simulink model "LundellAlternatorDC"  (R2018a)
settings: Solver=VariableStepAuto  StartTime=0  StopTime=0.2  FixedStep=1e-6
undefined symbols (not defined in the file): alternator, i_f_max, n_r, rectifier, T_s, v_dc_ref
libraries: fl_lib x32, nesl_utility x31, elec_lib x20, powerlib_meascontrol x6, SimscapeCustomBlocks_lib x2
settings Model: Creator=gabrielrodrigues  LastModifiedBy=gabrielrodrigues
settings DataIOCC: ReturnWorkspaceOutputs=on
settings CodeAppCC: StateflowObjectComments=on
settings SimscapeCC: SimscapeNormalizeSystem=off  SimscapeLogType=local  SimscapeLogLimitData=off

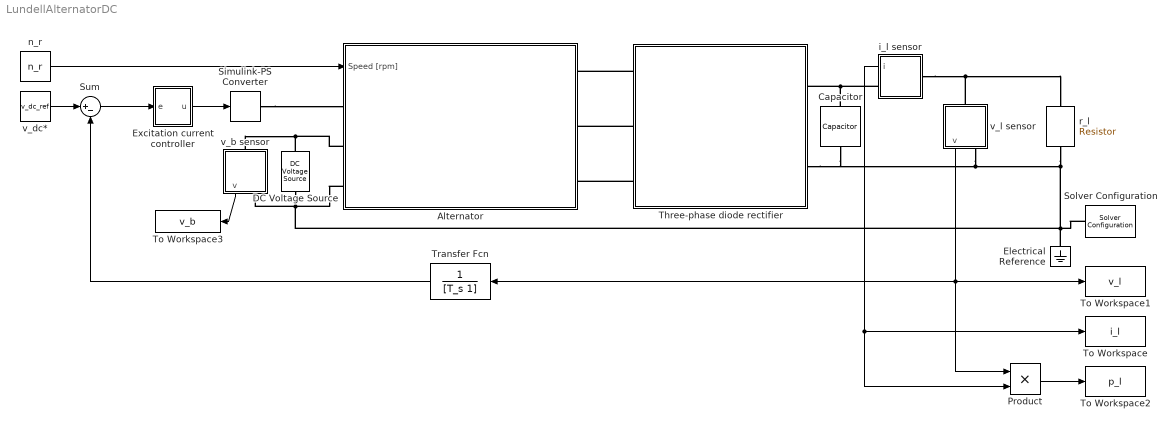
== system LundellAlternatorDC ==
  Alternator : Subsystem
  Capacitor : fl_lib/Electrical/Electrical Elements/Capacitor  c=rectifier.filter.c F  r=1e-6 Ohm  g=0 1/Ohm  i_specify=off  i_priority=None  i=0 A  i_nominal_specify=off  i_nominal_unit=A  i_nominal_value=1  v_specify=off  v_priority=None  v=0 V  v_nominal_specify=off  v_nominal_unit=V  v_nominal_value=1  vc_specify=off  vc_priority=High  vc=0 V  vc_nominal_specify=off  vc_nominal_unit=V  vc_nominal_value=1
  DC Voltage Source : elec_lib/Additional Components/SPICE-Compatible Components/Sources/DC Voltage Source  DC=i_f_max * alternator.rotor.r.value V
      settings: SourceProductName=Simscape Electronics  SourceProductBaseCode=SN
  Electrical Reference : fl_lib/Electrical/Electrical Elements/Electrical Reference
  Excitation current controller : Subsystem  mask{controller_on_off=Controller active}
      mask TypeOptions controller_on_off: Controller active | Controller bypassed
  Product : Product
  Simulink-PS Converter : nesl_utility/Simulink-PS Converter  PhysicalDomain=network_engine_domain  SubClassName=ps_input  LeftPortType=input  RightPortType=output  PseudoPeriodic=off  Frequencies=[]  NoiseDistribution=none  NoiseParameters=[]  Unit=1  AffineConversion=off  FilteringAndDerivatives=provide  SimscapeFilterOrder=1  InputFilterTimeConstant=0.001  UdotUserProvided=0
  Solver Configuration : nesl_utility/Solver Configuration  PhysicalDomain=network_engine_domain  SubClassName=solver  LeftPortType=input  RightPortType=generic  Tones=[]  Harmonics=[]  SimulateNoise=off  Profile=off  UseLocalSampling=off  EnableSwitchedLinearOptims=on  FrequencyDomain=off  UseCCode=off  RelTol=0.001  AbsTol=1e-06  MinStep=1e-09  ToWorkspace=off  RevertToSquareIcSolve=off  NumHomotopyIterations=100  PhasorMode=off  PhasorModeNumHarmonics=1  DoDC=off  ResidualTolerance=1e-09  UseLocalSolver=on  LocalSolverChoice=NE_TRAPEZOIDAL_ADVANCER  LocalSolverSampleTime=1e-06  DoFixedCost=on  MaxNonlinIter=20  MaxModeIter=2  LinearAlgebra=Sparse  EquationFormulation=NE_TIME_EF  DelaysMemoryBudget=1024  AutomaticFiltering=on  FilteringTimeConstant=0.001
  Sum : Sum  Inputs=|+-
  Three-phase diode rectifier : Subsystem
  To Workspace : ToWorkspace  VariableName=i_l  SaveFormat=Timeseries  SampleTime=-1
  To Workspace1 : ToWorkspace  VariableName=v_l  SaveFormat=Timeseries  SampleTime=-1
  To Workspace2 : ToWorkspace  VariableName=p_l  SaveFormat=Timeseries  SampleTime=-1
  To Workspace3 : ToWorkspace  VariableName=v_b  SaveFormat=Timeseries  SampleTime=-1
  Transfer Fcn : TransferFcn  Denominator=[T_s 1]
  i_l sensor : Subsystem
  n_r : Constant  Value=n_r
  r_l : fl_lib/Electrical/Electrical Elements/Resistor  R=1.0 Ohm  i_specify=off  i_priority=None  i=0 A  i_nominal_specify=off  i_nominal_unit=A  i_nominal_value=1  v_specify=off  v_priority=None  v=0 V  v_nominal_specify=off  v_nominal_unit=V  v_nominal_value=1
  v_b sensor : Subsystem
  v_dc* : Constant  Value=v_dc_ref
  v_l sensor : Subsystem
  wires:
  n_r/1 -> Alternator/1(Speed [rpm])
  Product/1 -> To Workspace2/1
  v_l sensor/1(v) -> Transfer Fcn/1, Product/1, To Workspace1/1
  v_b sensor/1(v) -> To Workspace3/1
  v_dc*/1 -> Sum/1
  Sum/1 -> Excitation current controller/1(e)
  Excitation current controller/1(u) -> Simulink-PS Converter/1
  Transfer Fcn/1 -> Sum/2
  i_l sensor/1(i) -> Product/2, To Workspace/1
  connections:
  Three-phase diode rectifier/LConn2 -- Alternator/RConn2
  Three-phase diode rectifier/LConn3 -- Alternator/RConn3
  Three-phase diode rectifier/LConn1 -- Alternator/RConn1
  i_l sensor/LConn1 -- r_l/LConn1 -- v_l sensor/LConn1
  v_b sensor/LConn1 -- DC Voltage Source/LConn1 -- Alternator/LConn2
  Solver Configuration/RConn1 -- DC Voltage Source/RConn1 -- Alternator/LConn3 -- v_b sensor/RConn1 -- Electrical Reference/LConn1 -- r_l/RConn1 -- Three-phase diode rectifier/RConn2 -- Capacitor/RConn1 -- v_l sensor/RConn1
  Simulink-PS Converter/RConn1 -- Alternator/LConn1
  i_l sensor/RConn1 -- Capacitor/LConn1 -- Three-phase diode rectifier/RConn1

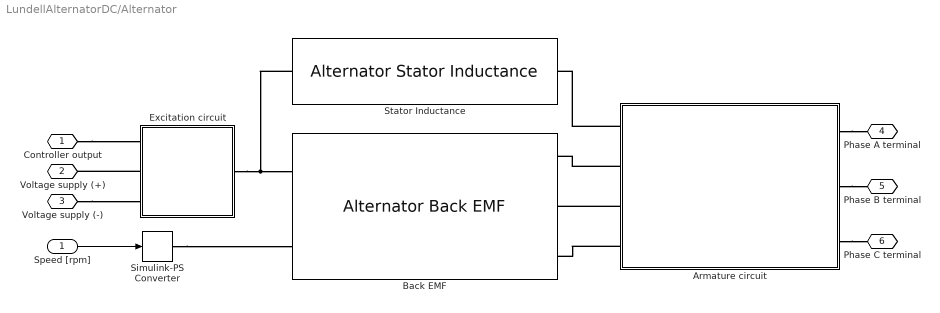
== system LundellAlternatorDC/Alternator ==
  Speed [rpm] : Inport
  Armature circuit : Subsystem  Variant=on
  Back EMF : SimscapeCustomBlocks_lib/Alternator/Alternator Back EMF  p=alternator.p  omega_r_specify=off  omega_r_priority=None  omega_r=0 rad/s  omega_r_nominal_specify=off  omega_r_nominal_unit=rad/s  omega_r_nominal_value=1  omega_e_specify=off  omega_e_priority=None  omega_e=0 rad/s  omega_e_nominal_specify=off  omega_e_nominal_unit=rad/s  omega_e_nominal_value=1  theta_e_specify=off  theta_e_priority=None  theta_e=0 rad  theta_e_nominal_specify=off  theta_e_nominal_unit=rad  theta_e_nominal_value=1  k_e_specify=off  k_e_priority=None  k_e=0 s*V/rad/A  k_e_nominal_specify=off  k_e_nominal_unit=s*V/rad/A  k_e_nominal_value=1  e_specify=off  e_priority=None  e=0 rpm  e_nominal_specify=off  e_nominal_unit=rpm  e_nominal_value=1
  Excitation circuit : Subsystem
  Simulink-PS Converter : nesl_utility/Simulink-PS Converter  PhysicalDomain=network_engine_domain  SubClassName=ps_input  LeftPortType=input  RightPortType=output  PseudoPeriodic=off  Frequencies=[]  NoiseDistribution=none  NoiseParameters=[]  Unit=1  AffineConversion=off  FilteringAndDerivatives=provide  SimscapeFilterOrder=1  InputFilterTimeConstant=0.001  UdotUserProvided=0
  Stator Inductance : SimscapeCustomBlocks_lib/Alternator/Alternator Stator Inductance
  Controller output : PMIOPort  Side=Left
  Voltage supply (+) : PMIOPort  Port=2  Side=Left
  Voltage supply (-) : PMIOPort  Port=3  Side=Left
  Phase A terminal : PMIOPort  Port=4  Side=Right
  Phase B terminal : PMIOPort  Port=5  Side=Right
  Phase C terminal : PMIOPort  Port=6  Side=Right
  wires:
  Speed [rpm]/1 -> Simulink-PS Converter/1
  connections:
  Armature circuit/RConn1 -- Phase A terminal/RConn1
  Armature circuit/RConn2 -- Phase B terminal/RConn1
  Armature circuit/RConn3 -- Phase C terminal/RConn1
  Armature circuit/LConn3 -- Back EMF/RConn2
  Armature circuit/LConn2 -- Back EMF/RConn1
  Armature circuit/LConn4 -- Back EMF/RConn3
  Simulink-PS Converter/RConn1 -- Back EMF/LConn2
  Armature circuit/LConn1 -- Stator Inductance/RConn1
  Controller output/RConn1 -- Excitation circuit/LConn1
  Voltage supply (-)/RConn1 -- Excitation circuit/LConn3
  Excitation circuit/LConn2 -- Voltage supply (+)/RConn1
  Excitation circuit/RConn1 -- Stator Inductance/LConn1 -- Back EMF/LConn1

== system LundellAlternatorDC/Excitation current controller ==
  e : Inport
  Constant : Constant
  Constant1 : Constant  Value=controller_on_off
  Fcn : Fcn  Expr=u > 0
  Switch : Switch  Criteria=u2 > Threshold  Threshold=1.5
  To Workspace : ToWorkspace  VariableName=u_i_f  SaveFormat=Timeseries  SampleTime=-1
  u : Outport
  wires:
  e/1 -> Fcn/1
  Fcn/1 -> Switch/3
  Switch/1 -> To Workspace/1, u/1
  Constant1/1 -> Switch/2
  Constant/1 -> Switch/1

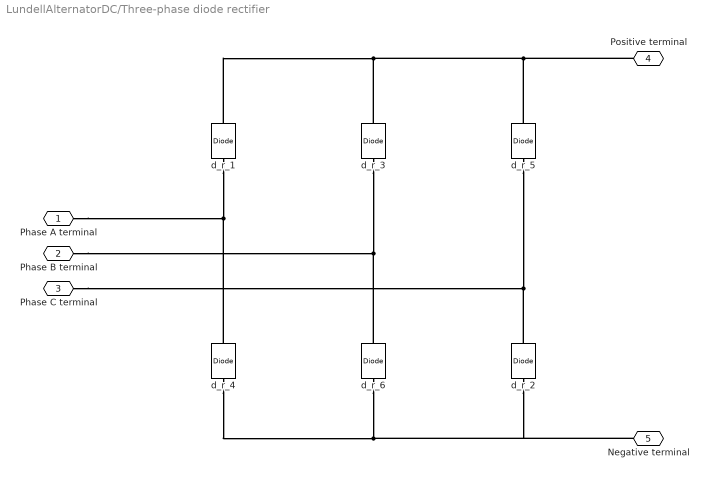
== system LundellAlternatorDC/Three-phase diode rectifier ==
  d_r_{1..6} (6 alike) : elec_lib/Semiconductor Devices/Diode  ModelType=1  Vf=rectifier.d.v_on V  Ron=rectifier.d.r_on Ohm  Goff=1e-8 S  Rz=0.3 Ohm  Vz=50 V  C_PWL=5 pF  prmExp=1  I12=[.0137, .545] A  V12=[.6, .7] V  I1=0.0137 A  V1=0.6 V  IS=1e-12 A  ec=1  RS=10e-3 Ohm  Tmeas=25 degC  BV=inf V  C_param=1  CJ0=5 pF  VJ=1 V  Mgrad=0.5  Vvec=[.1, 10, 100] V  Cvec=[3.5, 1, .4] pF  FC=0.5  Q_param=1  Irrm=-7.15 A  iF=4 A  didt=-750 A/us  trr=115 ns  TT=50 ns  tau=100 ns  T_param=1  IS_T2=1.25e-7 A  I1_T2=0.245 A  V1_T2=0.5 V  Tmeas2=125 degC  EG_param=1  EG=1.11 eV  XTI_param=1  XTI=3  dBVdT=0 V/K  Tdevice=25 degC  i_capacitor_specify=off  i_capacitor_priority=High  i_capacitor=0 A  i_capacitor_nominal_specify=off  i_capacitor_nominal_unit=A  i_capacitor_nominal_value=1  v_capacitor_specify=off  v_capacitor_priority=None  v_capacitor=0 V  v_capacitor_nominal_specify=off  v_capacitor_nominal_unit=V  v_capacitor_nominal_value=1  Rth=[0, 10] K/W  thermal_mass_parameterization=1  thermal_mass=[0, 1] J/K  thermal_time_constant=[0, 10] s  thermal_mass_initial_temperatures=[25, 25] degC
      settings: SourceProductName=Simscape Electronics  SourceProductBaseCode=SN
  Phase A terminal : PMIOPort  Side=Left
  Phase B terminal : PMIOPort  Port=2  Side=Left
  Phase C terminal : PMIOPort  Port=3  Side=Left
  Positive terminal : PMIOPort  Port=4  Side=Right
  Negative terminal : PMIOPort  Port=5  Side=Right
  connections:
  Phase B terminal/RConn1 -- d_r_6/RConn1 -- d_r_3/LConn1
  Positive terminal/RConn1 -- d_r_5/RConn1 -- d_r_1/RConn1 -- d_r_3/RConn1
  d_r_1/LConn1 -- Phase A terminal/RConn1 -- d_r_4/RConn1
  Phase C terminal/RConn1 -- d_r_5/LConn1 -- d_r_2/RConn1
  d_r_2/LConn1 -- Negative terminal/RConn1 -- d_r_6/LConn1 -- d_r_4/LConn1

== system LundellAlternatorDC/i_l sensor ==
  Current Sensor : fl_lib/Electrical/Electrical Sensors/Current Sensor
  PS-Simulink Converter : nesl_utility/PS-Simulink Converter  PhysicalDomain=network_engine_domain  SubClassName=ps_output  LeftPortType=input  RightPortType=output  PseudoPeriodic=off  Frequencies=[]  Unit=1  AffineConversion=off
  + : PMIOPort  Side=Right
  - : PMIOPort  Port=2  Side=Left
  i : Outport
  wires:
  PS-Simulink Converter/1 -> i/1
  connections:
  Current Sensor/RConn2 -- -/RConn1
  Current Sensor/LConn1 -- +/RConn1
  PS-Simulink Converter/LConn1 -- Current Sensor/RConn1

== system LundellAlternatorDC/v_b sensor ==
  PS-Simulink Converter : nesl_utility/PS-Simulink Converter  PhysicalDomain=network_engine_domain  SubClassName=ps_output  LeftPortType=input  RightPortType=output  PseudoPeriodic=off  Frequencies=[]  Unit=1  AffineConversion=off
  Voltage Sensor : fl_lib/Electrical/Electrical Sensors/Voltage Sensor
  + : PMIOPort  Side=Left
  - : PMIOPort  Port=2  Side=Right
  v : Outport
  wires:
  PS-Simulink Converter/1 -> v/1
  connections:
  Voltage Sensor/LConn1 -- +/RConn1
  -/RConn1 -- Voltage Sensor/RConn2
  Voltage Sensor/RConn1 -- PS-Simulink Converter/LConn1

== system LundellAlternatorDC/v_l sensor ==
  PS-Simulink Converter : nesl_utility/PS-Simulink Converter  PhysicalDomain=network_engine_domain  SubClassName=ps_output  LeftPortType=input  RightPortType=output  PseudoPeriodic=off  Frequencies=[]  Unit=1  AffineConversion=off
  Voltage Sensor : fl_lib/Electrical/Electrical Sensors/Voltage Sensor
  + : PMIOPort  Side=Left
  - : PMIOPort  Port=2  Side=Right
  v : Outport
  wires:
  PS-Simulink Converter/1 -> v/1
  connections:
  Voltage Sensor/LConn1 -- +/RConn1
  -/RConn1 -- Voltage Sensor/RConn2
  Voltage Sensor/RConn1 -- PS-Simulink Converter/LConn1

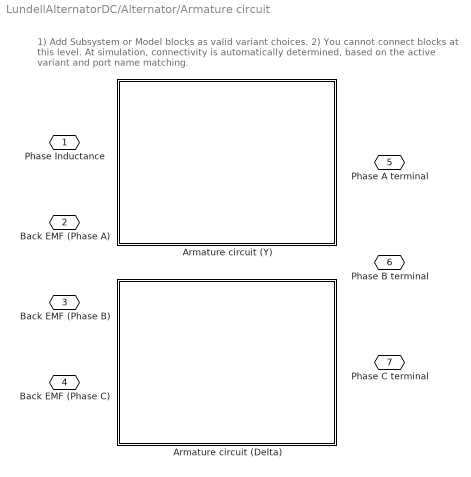
== system LundellAlternatorDC/Alternator/Armature circuit ==
  note: 1) Add Subsystem or Model blocks as valid variant choices.
      | 2) You cannot connect blocks at this level. At simulation, connectivity is automatically
      | determined, based on the active variant and port name matching.
  Armature circuit (Delta) : Subsystem  VariantControl=deltaStatorConnection
  Armature circuit (Y) : Subsystem  VariantControl=yStatorConnection
  Phase Inductance : PMIOPort  Side=Left
  Back EMF (Phase A) : PMIOPort  Port=2  Side=Left
  Back EMF (Phase B) : PMIOPort  Port=3  Side=Left
  Back EMF (Phase C) : PMIOPort  Port=4  Side=Left
  Phase A terminal : PMIOPort  Port=5  Side=Right
  Phase B terminal : PMIOPort  Port=6  Side=Right
  Phase C terminal : PMIOPort  Port=7  Side=Right

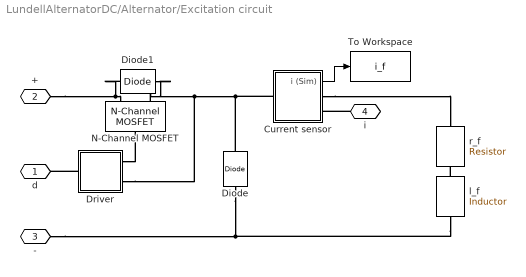
== system LundellAlternatorDC/Alternator/Excitation circuit ==
  Current sensor : Subsystem
  Diode : elec_lib/Semiconductor Devices/Diode  ModelType=1  Vf=0.8 V  Ron=10e-3 Ohm  Goff=1e-8 S  Rz=0.3 Ohm  Vz=50 V  C_PWL=5 pF  prmExp=1  I12=[.0137, .545] A  V12=[.6, .7] V  I1=0.0137 A  V1=0.6 V  IS=1e-12 A  ec=1  RS=10e-3 Ohm  Tmeas=25 degC  BV=inf V  C_param=1  CJ0=5 pF  VJ=1 V  Mgrad=0.5  Vvec=[.1, 10, 100] V  Cvec=[3.5, 1, .4] pF  FC=0.5  Q_param=1  Irrm=-7.15 A  iF=4 A  didt=-750 A/us  trr=115 ns  TT=50 ns  tau=100 ns  T_param=1  IS_T2=1.25e-7 A  I1_T2=0.245 A  V1_T2=0.5 V  Tmeas2=125 degC  EG_param=1  EG=1.11 eV  XTI_param=1  XTI=3  dBVdT=0 V/K  Tdevice=25 degC  i_capacitor_specify=off  i_capacitor_priority=High  i_capacitor=0 A  i_capacitor_nominal_specify=off  i_capacitor_nominal_unit=A  i_capacitor_nominal_value=1  v_capacitor_specify=off  v_capacitor_priority=None  v_capacitor=0 V  v_capacitor_nominal_specify=off  v_capacitor_nominal_unit=V  v_capacitor_nominal_value=1  Rth=[0, 10] K/W  thermal_mass_parameterization=1  thermal_mass=[0, 1] J/K  thermal_time_constant=[0, 10] s  thermal_mass_initial_temperatures=[25, 25] degC
      settings: SourceProductName=Simscape Electronics  SourceProductBaseCode=SN
  Diode1 : elec_lib/Semiconductor Devices/Diode  ModelType=1  Vf=0.8 V  Ron=10e-3 Ohm  Goff=1e-8 S  Rz=0.3 Ohm  Vz=50 V  C_PWL=5 pF  prmExp=1  I12=[.0137, .545] A  V12=[.6, .7] V  I1=0.0137 A  V1=0.6 V  IS=1e-12 A  ec=1  RS=10e-3 Ohm  Tmeas=25 degC  BV=inf V  C_param=1  CJ0=5 pF  VJ=1 V  Mgrad=0.5  Vvec=[.1, 10, 100] V  Cvec=[3.5, 1, .4] pF  FC=0.5  Q_param=1  Irrm=-7.15 A  iF=4 A  didt=-750 A/us  trr=115 ns  TT=50 ns  tau=100 ns  T_param=1  IS_T2=1.25e-7 A  I1_T2=0.245 A  V1_T2=0.5 V  Tmeas2=125 degC  EG_param=1  EG=1.11 eV  XTI_param=1  XTI=3  dBVdT=0 V/K  Tdevice=25 degC  i_capacitor_specify=off  i_capacitor_priority=High  i_capacitor=0 A  i_capacitor_nominal_specify=off  i_capacitor_nominal_unit=A  i_capacitor_nominal_value=1  v_capacitor_specify=off  v_capacitor_priority=None  v_capacitor=0 V  v_capacitor_nominal_specify=off  v_capacitor_nominal_unit=V  v_capacitor_nominal_value=1  Rth=[0, 10] K/W  thermal_mass_parameterization=1  thermal_mass=[0, 1] J/K  thermal_time_constant=[0, 10] s  thermal_mass_initial_temperatures=[25, 25] degC
      settings: SourceProductName=Simscape Electronics  SourceProductBaseCode=SN
  Driver : Subsystem
  N-Channel MOSFET : elec_lib/Semiconductor Devices/N-Channel MOSFET  parameterization=1  prmDatasheet=1  prmEquCoeff=1  Beta=5 A/V^2  Rds=0.025 Ohm  Id=6 A  Vgs=alternator.rotor.s.v_gs_on V  Vth=1.7 V  lam=0 1/V  Tmeas=25 degC  RS=1e-4 Ohm  RD=0.01 Ohm  C_param=1  C_GS=270 pF  C_GD=80 pF  C_DS=0 pF  C_iss=350 pF  C_rss=80 pF  C_oss=0 pF  C_GS_vec=[ 270 300 290 280 295 255 ] pF  C_GD_vec=[ 450 400 300 190 95 55 ] pF  C_DS_vec=[ 450 410 390 230 175 115 ] pF  C_iss_vec=[ 720 700 590 470 390 310 ] pF  C_rss_vec=[ 450 400 300 190 95 55 ] pF  C_oss_vec=[ 900 810 690 420 270 170 ] pF  C_Vds_vec=[ 0.1 0.3 1 3 10 30 ] V  V_GS_for_cap_data=0 V  charge_linearity_param=1  C_OX=200 pF  V_C_OX=-0.5 V  IsDiode=0 A  Vbi=0.6 V  n=1  Cj0Diode=0 pF  TT=50e-9 s  dVth_dT=-6 mV/K  Rds_T2=0.037 Ohm  Tmeas2=125 degC  BEXDatasheet=-1.5  BEXEquCoeff=-1.5  etaisDatasheet=3  etaisEquCoeff=3  TdeviceDatasheet=25 degC  TdeviceEquCoeff=25 degC  Rth=[1, 10] K/W  thermal_mass_parameterization=1  thermal_mass=[1, 1] J/K  thermal_time_constant=[1, 10] s  thermal_mass_initial_temperatures=[ 25 25 ] degC  betaref=18 A/V^2  Vfbref=-1.1 V  gamma=3.5 V^0.50000  phib2ref=1 V  thesatref=0.4 1/V  alpha=0  Vp=5e-2 V  thesrref=0 1/V  m=8  Tref=25 degC  Cox=1500 pF  Cgso=100 pF  Cgdo=14 pF  Rsref=2e-3 Ohm  Rdref=0.17 Ohm  Rgref=8.4 Ohm  Isref=5.2e-13 A  Cj0=480 pF  Tprm=1  etabet=1.3  Stvfb=5e-4 V/K  Stphib=-8.5e-4 V/K  etasat=1.04  etasr=0.65  etar=0.95  etais=3  Tsim=25 degC  T0=[25, 25] degC
      settings: SourceProductName=Simscape Electronics  SourceProductBaseCode=SN
  To Workspace : ToWorkspace  VariableName=i_f  SaveFormat=Timeseries  SampleTime=-1
  l_f : elec_lib/Passive Devices/Inductor  l=alternator.rotor.l.value H  L_tol=20  enable_L_tol=0  tol_distribution=1  nSigma=4  r=0 Ohm  g=1e-9 1/Ohm  enable_operating_limits=0  operating_limit_action=2  max_working_current=1 A  power_rating=1 W  enable_faults=0  fault_action=1  lambdaPercent=50  k_faulted=0.9999  turnsShort=0  openCct=0  groundShort=0  groundShortG=0 1/Ohm  tau_fault=1e-3 s  enable_temporal_fault=0  t_fault=1 s  enable_behavioral_fault=0  max_permissible_voltage=100 V  n_fail_on_voltage=1  max_permissible_current=1 A  t_fail_on_current=1 s  i_L_specify=off  i_L_priority=High  i_L=0 A  i_L_nominal_specify=off  i_L_nominal_unit=A  i_L_nominal_value=1
      settings: SourceProductName=Simscape Electronics  SourceProductBaseCode=SN
  r_f : elec_lib/Passive Devices/Resistor  R=alternator.rotor.r.value Ohm  R_tol=5  enable_R_tol=0  tol_distribution=1  nSigma=4  enable_operating_limits=0  operating_limit_action=2  max_working_voltage=100 V  power_rating=1 W  enable_faults=0  fault_action=1  R_faulted=inf Ohm  enable_temporal_fault=0  t_fault=1 s  enable_behavioral_fault=0  max_permissible_current=1 A  t_fail_on_current=1 s  noise_mode=0  sample_time=1e-3 s  repeatability=1  auto_seed=3032444857  user_seed=0  Tdevice=25 degC  alpha=3.93e-3 1/K  Tmeas=25 degC  thermal_mass=100 J/K  power_derating_T1=70 degC  power_derating_T2=155 degC  operating_temperature_range_vec=[-50.0, 150.0] degC  temperature_specify=off  temperature_priority=High  temperature=298.15 K  temperature_nominal_specify=off  temperature_nominal_unit=K  temperature_nominal_value=1
  d : PMIOPort  Side=Left
  + : PMIOPort  Port=2  Side=Left
  - : PMIOPort  Port=3  Side=Left
  i : PMIOPort  Port=4  Side=Right
  wires:
  Current sensor/1(i (Sim)) -> To Workspace/1
  connections:
  l_f/RConn1 -- Diode/LConn1 -- -/RConn1
  +/RConn1 -- Diode1/RConn1 -- N-Channel MOSFET/RConn1
  Current sensor/RConn1 -- r_f/RConn1
  Current sensor/LConn1 -- Diode/RConn1 -- Driver/RConn2 -- Diode1/LConn1 -- N-Channel MOSFET/RConn2
  l_f/LConn1 -- r_f/LConn1
  Driver/RConn1 -- N-Channel MOSFET/LConn1
  i/RConn1 -- Current sensor/RConn2
  Driver/LConn1 -- d/RConn1

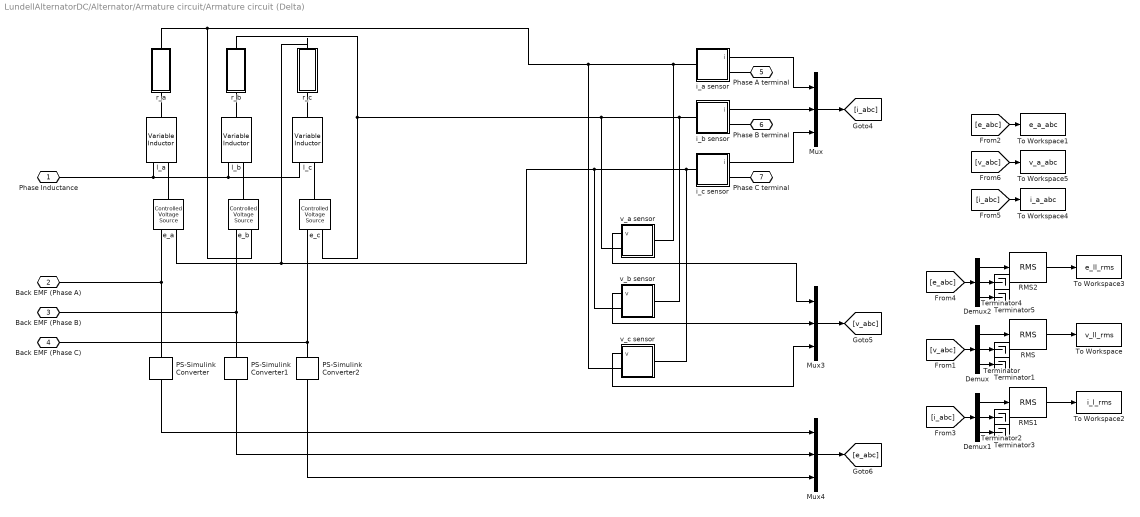
== system LundellAlternatorDC/Alternator/Armature circuit/Armature circuit (Delta) ==
  Demux : Demux  Outputs=3
  Demux1 : Demux  Outputs=3
  Demux2 : Demux  Outputs=3
  Mux : Mux  Inputs=3
  Mux3 : Mux  Inputs=3
  Mux4 : Mux  Inputs=3
  PS-Simulink Converter : nesl_utility/PS-Simulink Converter  PhysicalDomain=network_engine_domain  SubClassName=ps_output  LeftPortType=input  RightPortType=output  PseudoPeriodic=off  Frequencies=[]  Unit=1  AffineConversion=off
  PS-Simulink Converter1 : nesl_utility/PS-Simulink Converter  PhysicalDomain=network_engine_domain  SubClassName=ps_output  LeftPortType=input  RightPortType=output  PseudoPeriodic=off  Frequencies=[]  Unit=1  AffineConversion=off
  PS-Simulink Converter2 : nesl_utility/PS-Simulink Converter  PhysicalDomain=network_engine_domain  SubClassName=ps_output  LeftPortType=input  RightPortType=output  PseudoPeriodic=off  Frequencies=[]  Unit=1  AffineConversion=off
  RMS : powerlib_meascontrol/Measurements/RMS  TrueRMS=on  Freq=8*2000/60  RMSInit=120  Ts=0
      settings: SourceProductName=Simscape Electrical
  RMS1 : powerlib_meascontrol/Measurements/RMS  TrueRMS=on  Freq=8*2000/60  RMSInit=120  Ts=0
      settings: SourceProductName=Simscape Electrical
  RMS2 : powerlib_meascontrol/Measurements/RMS  TrueRMS=on  Freq=8*2000/60  RMSInit=120  Ts=0
      settings: SourceProductName=Simscape Electrical
  Terminator{,1..5} (6 alike) : Terminator
  To Workspace : ToWorkspace  VariableName=v_ll_rms  SaveFormat=Timeseries  SampleTime=-1
  To Workspace1 : ToWorkspace  VariableName=e_a_abc  SaveFormat=Timeseries  SampleTime=-1
  To Workspace2 : ToWorkspace  VariableName=i_l_rms  SaveFormat=Timeseries  SampleTime=-1
  To Workspace3 : ToWorkspace  VariableName=e_ll_rms  SaveFormat=Timeseries  SampleTime=-1
  To Workspace4 : ToWorkspace  VariableName=i_a_abc  SaveFormat=Timeseries  SampleTime=-1
  To Workspace5 : ToWorkspace  VariableName=v_a_abc  SaveFormat=Timeseries  SampleTime=-1
  e_a : fl_lib/Electrical/Electrical Sources/Controlled Voltage Source
  e_b : fl_lib/Electrical/Electrical Sources/Controlled Voltage Source
  e_c : fl_lib/Electrical/Electrical Sources/Controlled Voltage Source
  i_a sensor : Subsystem
  i_b sensor : Subsystem
  i_c sensor : Subsystem
  l_a : elec_lib/Passive Devices/Variable Inductor  prm=1  Lmin=1e-6 H  g=1e-9 1/Ohm  i0=0 A  phi0=0 Wb
      settings: SourceProductName=Simscape Electronics  SourceProductBaseCode=SN
  l_b : elec_lib/Passive Devices/Variable Inductor  prm=1  Lmin=1e-6 H  g=1e-9 1/Ohm  i0=0 A  phi0=0 Wb
      settings: SourceProductName=Simscape Electronics  SourceProductBaseCode=SN
  l_c : elec_lib/Passive Devices/Variable Inductor  prm=1  Lmin=1e-6 H  g=1e-9 1/Ohm  i0=0 A  phi0=0 Wb
      settings: SourceProductName=Simscape Electronics  SourceProductBaseCode=SN
  r_a : Subsystem  mask{r_ref=alternator.stator.r.value, T_ref=alternator.stator.r.T_ref, T=alternator.stator.r.T, alpha=alternator.stator.r.alpha}
      mask prompts: r_ref "Nominal resistance [Ohm]"; T_ref "Reference temperature [oC]"; T "Resistor temperature [oC]"; alpha "Temperature Coefficient [1/oC]"
  r_b : Subsystem  mask{r_ref=alternator.stator.r.value, T_ref=alternator.stator.r.T_ref, T=alternator.stator.r.T, alpha=alternator.stator.r.alpha}
      mask prompts: r_ref "Nominal resistance [Ohm]"; T_ref "Reference temperature [oC]"; T "Resistor temperature [oC]"; alpha "Temperature Coefficient [1/oC]"
  r_c : Subsystem  mask{r_ref=alternator.stator.r.value, T_ref=alternator.stator.r.T_ref, T=alternator.stator.r.T, alpha=alternator.stator.r.alpha}
      mask prompts: r_ref "Nominal resistance [Ohm]"; T_ref "Reference temperature [oC]"; T "Resistor temperature [oC]"; alpha "Temperature Coefficient [1/oC]"
  v_a sensor : Subsystem
  v_b sensor : Subsystem
  v_c sensor : Subsystem
  Phase Inductance : PMIOPort  Side=Left
  Back EMF (Phase A) : PMIOPort  Port=2  Side=Left
  Back EMF (Phase B) : PMIOPort  Port=3  Side=Left
  Back EMF (Phase C) : PMIOPort  Port=4  Side=Left
  Phase A terminal : PMIOPort  Port=5  Side=Right
  Phase B terminal : PMIOPort  Port=6  Side=Right
  Phase C terminal : PMIOPort  Port=7  Side=Right
  wires:
  i_a sensor/1(i) -> Mux/1
  i_b sensor/1(i) -> Mux/2
  i_c sensor/1(i) -> Mux/3
  Mux/1 -> [i_abc]
  Mux3/1 -> [v_abc]
  v_b sensor/1(v) -> Mux3/2
  v_c sensor/1(v) -> Mux3/3
  v_a sensor/1(v) -> Mux3/1
  PS-Simulink Converter/1 -> Mux4/1
  PS-Simulink Converter1/1 -> Mux4/2
  PS-Simulink Converter2/1 -> Mux4/3
  Mux4/1 -> [e_abc]
  Demux/3 -> Terminator1/1
  Demux/2 -> Terminator/1
  Demux2/2 -> Terminator4/1
  [e_abc] -> Demux2/1
  RMS2/1 -> To Workspace3/1
  Demux2/1 -> RMS2/1
  Demux2/3 -> Terminator5/1
  Demux1/2 -> Terminator2/1
  [e_abc] -> To Workspace1/1
  RMS/1 -> To Workspace/1
  Demux/1 -> RMS/1
  RMS1/1 -> To Workspace2/1
  [i_abc] -> Demux1/1
  [v_abc] -> Demux/1
  Demux1/3 -> Terminator3/1
  [v_abc] -> To Workspace5/1
  Demux1/1 -> RMS1/1
  [i_abc] -> To Workspace4/1
  connections:
  i_a sensor/RConn1 -- Phase A terminal/RConn1
  Back EMF (Phase A)/RConn1 -- e_a/RConn1 -- PS-Simulink Converter/LConn1
  Back EMF (Phase B)/RConn1 -- e_b/RConn1 -- PS-Simulink Converter1/LConn1
  Back EMF (Phase C)/RConn1 -- e_c/RConn1 -- PS-Simulink Converter2/LConn1
  e_c/LConn1 -- l_c/LConn2
  e_b/LConn1 -- l_b/LConn2
  e_a/LConn1 -- l_a/LConn2
  r_c/LConn1 -- l_c/RConn1
  r_b/LConn1 -- l_b/RConn1
  r_a/LConn1 -- l_a/RConn1
  i_c sensor/RConn1 -- Phase C terminal/RConn1
  i_b sensor/RConn1 -- Phase B terminal/RConn1
  l_a/LConn1 -- Phase Inductance/RConn1 -- l_b/LConn1 -- l_c/LConn1
  e_b/RConn2 -- v_a sensor/LConn1 -- i_a sensor/LConn1 -- v_c sensor/RConn1 -- r_a/RConn1
  v_a sensor/RConn1 -- i_b sensor/LConn1 -- v_b sensor/LConn1 -- e_c/RConn2 -- r_b/RConn1
  e_a/RConn2 -- v_c sensor/LConn1 -- i_c sensor/LConn1 -- v_b sensor/RConn1 -- r_c/RConn1

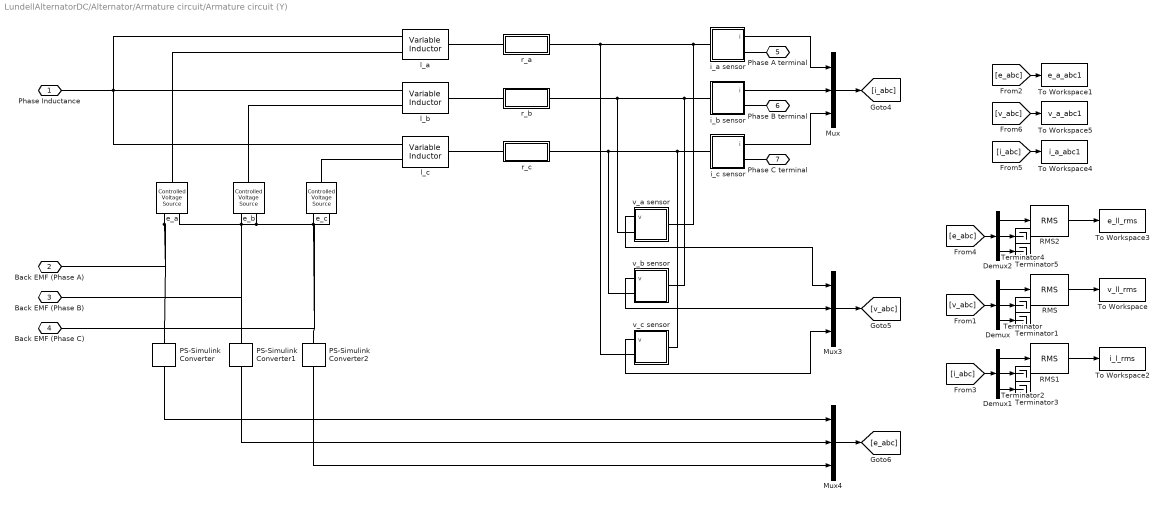
== system LundellAlternatorDC/Alternator/Armature circuit/Armature circuit (Y) ==
  Demux : Demux  Outputs=3
  Demux1 : Demux  Outputs=3
  Demux2 : Demux  Outputs=3
  Mux : Mux  Inputs=3
  Mux3 : Mux  Inputs=3
  Mux4 : Mux  Inputs=3
  PS-Simulink Converter : nesl_utility/PS-Simulink Converter  PhysicalDomain=network_engine_domain  SubClassName=ps_output  LeftPortType=input  RightPortType=output  PseudoPeriodic=off  Frequencies=[]  Unit=1  AffineConversion=off
  PS-Simulink Converter1 : nesl_utility/PS-Simulink Converter  PhysicalDomain=network_engine_domain  SubClassName=ps_output  LeftPortType=input  RightPortType=output  PseudoPeriodic=off  Frequencies=[]  Unit=1  AffineConversion=off
  PS-Simulink Converter2 : nesl_utility/PS-Simulink Converter  PhysicalDomain=network_engine_domain  SubClassName=ps_output  LeftPortType=input  RightPortType=output  PseudoPeriodic=off  Frequencies=[]  Unit=1  AffineConversion=off
  RMS : powerlib_meascontrol/Measurements/RMS  TrueRMS=on  Freq=8*2000/60  RMSInit=120  Ts=0
      settings: SourceProductName=Simscape Electrical
  RMS1 : powerlib_meascontrol/Measurements/RMS  TrueRMS=on  Freq=8*2000/60  RMSInit=120  Ts=0
      settings: SourceProductName=Simscape Electrical
  RMS2 : powerlib_meascontrol/Measurements/RMS  TrueRMS=on  Freq=8*2000/60  RMSInit=120  Ts=0
      settings: SourceProductName=Simscape Electrical
  Terminator{,1..5} (6 alike) : Terminator
  To Workspace : ToWorkspace  VariableName=v_ll_rms  SaveFormat=Timeseries  SampleTime=-1
  To Workspace1 : ToWorkspace  VariableName=e_a_abc1  SaveFormat=Timeseries  SampleTime=-1
  To Workspace2 : ToWorkspace  VariableName=i_l_rms  SaveFormat=Timeseries  SampleTime=-1
  To Workspace3 : ToWorkspace  VariableName=e_ll_rms  SaveFormat=Timeseries  SampleTime=-1
  To Workspace4 : ToWorkspace  VariableName=i_a_abc1  SaveFormat=Timeseries  SampleTime=-1
  To Workspace5 : ToWorkspace  VariableName=v_a_abc1  SaveFormat=Timeseries  SampleTime=-1
  e_a : fl_lib/Electrical/Electrical Sources/Controlled Voltage Source
  e_b : fl_lib/Electrical/Electrical Sources/Controlled Voltage Source
  e_c : fl_lib/Electrical/Electrical Sources/Controlled Voltage Source
  i_a sensor : Subsystem
  i_b sensor : Subsystem
  i_c sensor : Subsystem
  l_a : elec_lib/Passive Devices/Variable Inductor  prm=1  Lmin=1e-6 H  g=1e-9 1/Ohm  i0=0 A  phi0=0 Wb
      settings: SourceProductName=Simscape Electronics  SourceProductBaseCode=SN
  l_b : elec_lib/Passive Devices/Variable Inductor  prm=1  Lmin=1e-6 H  g=1e-9 1/Ohm  i0=0 A  phi0=0 Wb
      settings: SourceProductName=Simscape Electronics  SourceProductBaseCode=SN
  l_c : elec_lib/Passive Devices/Variable Inductor  prm=1  Lmin=1e-6 H  g=1e-9 1/Ohm  i0=0 A  phi0=0 Wb
      settings: SourceProductName=Simscape Electronics  SourceProductBaseCode=SN
  r_a : Subsystem  mask{r_ref=alternator.stator.r.value, T_ref=alternator.stator.r.T_ref, T=alternator.stator.r.T, alpha=alternator.stator.r.alpha}
      mask prompts: r_ref "Nominal resistance [Ohm]"; T_ref "Reference temperature [oC]"; T "Resistor temperature [oC]"; alpha "Temperature Coefficient [1/oC]"
  r_b : Subsystem  mask{r_ref=alternator.stator.r.value, T_ref=alternator.stator.r.T_ref, T=alternator.stator.r.T, alpha=alternator.stator.r.alpha}
      mask prompts: r_ref "Nominal resistance [Ohm]"; T_ref "Reference temperature [oC]"; T "Resistor temperature [oC]"; alpha "Temperature Coefficient [1/oC]"
  r_c : Subsystem  mask{r_ref=alternator.stator.r.value, T_ref=alternator.stator.r.T_ref, T=alternator.stator.r.T, alpha=alternator.stator.r.alpha}
      mask prompts: r_ref "Nominal resistance [Ohm]"; T_ref "Reference temperature [oC]"; T "Resistor temperature [oC]"; alpha "Temperature Coefficient [1/oC]"
  v_a sensor : Subsystem
  v_b sensor : Subsystem
  v_c sensor : Subsystem
  Phase Inductance : PMIOPort  Side=Left
  Back EMF (Phase A) : PMIOPort  Port=2  Side=Left
  Back EMF (Phase B) : PMIOPort  Port=3  Side=Left
  Back EMF (Phase C) : PMIOPort  Port=4  Side=Left
  Phase A terminal : PMIOPort  Port=5  Side=Right
  Phase B terminal : PMIOPort  Port=6  Side=Right
  Phase C terminal : PMIOPort  Port=7  Side=Right
  wires:
  i_a sensor/1(i) -> Mux/1
  i_b sensor/1(i) -> Mux/2
  i_c sensor/1(i) -> Mux/3
  Mux/1 -> [i_abc]
  Mux3/1 -> [v_abc]
  v_b sensor/1(v) -> Mux3/2
  v_c sensor/1(v) -> Mux3/3
  v_a sensor/1(v) -> Mux3/1
  PS-Simulink Converter/1 -> Mux4/1
  PS-Simulink Converter1/1 -> Mux4/2
  PS-Simulink Converter2/1 -> Mux4/3
  Mux4/1 -> [e_abc]
  Demux/3 -> Terminator1/1
  Demux/2 -> Terminator/1
  Demux2/2 -> Terminator4/1
  [e_abc] -> Demux2/1
  RMS2/1 -> To Workspace3/1
  Demux2/1 -> RMS2/1
  Demux2/3 -> Terminator5/1
  Demux1/2 -> Terminator2/1
  [e_abc] -> To Workspace1/1
  RMS/1 -> To Workspace/1
  Demux/1 -> RMS/1
  RMS1/1 -> To Workspace2/1
  [i_abc] -> Demux1/1
  [v_abc] -> Demux/1
  Demux1/3 -> Terminator3/1
  [v_abc] -> To Workspace5/1
  Demux1/1 -> RMS1/1
  [i_abc] -> To Workspace4/1
  connections:
  i_a sensor/RConn1 -- Phase A terminal/RConn1
  e_a/RConn2 -- e_c/RConn2 -- e_b/RConn2
  e_c/LConn1 -- l_c/LConn2
  e_b/LConn1 -- l_b/LConn2
  e_a/LConn1 -- l_a/LConn2
  r_c/LConn1 -- l_c/RConn1
  r_b/LConn1 -- l_b/RConn1
  r_a/LConn1 -- l_a/RConn1
  i_a sensor/LConn1 -- v_a sensor/LConn1 -- v_c sensor/RConn1 -- r_a/RConn1
  i_c sensor/RConn1 -- Phase C terminal/RConn1
  i_b sensor/RConn1 -- Phase B terminal/RConn1
  i_c sensor/LConn1 -- v_c sensor/LConn1 -- v_b sensor/RConn1 -- r_c/RConn1
  v_a sensor/RConn1 -- v_b sensor/LConn1 -- i_b sensor/LConn1 -- r_b/RConn1
  l_a/LConn1 -- Phase Inductance/RConn1 -- l_c/LConn1 -- l_b/LConn1
  e_a/RConn1 -- Back EMF (Phase A)/RConn1 -- PS-Simulink Converter/LConn1
  e_b/RConn1 -- Back EMF (Phase B)/RConn1 -- PS-Simulink Converter1/LConn1
  e_c/RConn1 -- Back EMF (Phase C)/RConn1 -- PS-Simulink Converter2/LConn1

== system LundellAlternatorDC/Alternator/Excitation circuit/Current sensor ==
  Current Sensor1 : fl_lib/Electrical/Electrical Sensors/Current Sensor
  PS-Simulink Converter1 : nesl_utility/PS-Simulink Converter  PhysicalDomain=network_engine_domain  SubClassName=ps_output  LeftPortType=input  RightPortType=output  PseudoPeriodic=off  Frequencies=[]  Unit=1  AffineConversion=off
  + : PMIOPort  Side=Left
  - : PMIOPort  Port=2  Side=Right
  i (PS) : PMIOPort  Port=3  Side=Right
  i (Sim) : Outport
  wires:
  PS-Simulink Converter1/1 -> i (Sim)/1
  connections:
  Current Sensor1/RConn2 -- -/RConn1
  Current Sensor1/LConn1 -- +/RConn1
  PS-Simulink Converter1/LConn1 -- i (PS)/RConn1 -- Current Sensor1/RConn1

== system LundellAlternatorDC/Alternator/Excitation circuit/Driver ==
  Controlled PWM Voltage : elec_lib/Actuators & Drivers/Drivers/Controlled PWM Voltage  F=alternator.rotor.control.pwm.f_s Hz  TD=0 s  pulse_width_offset=0 s  pulse_min=0 s  Vmin=0 V  Vmax=5 V  Vm=5 V  pwm_or_av=1  event_type=2  sample_time=T_s s  u_min=0  u_max=1
      settings: SourceProductName=Simscape Electronics  SourceProductBaseCode=SN  LogSimulationData=on
  Electrical Reference : fl_lib/Electrical/Electrical Elements/Electrical Reference
  Gate Driver : elec_lib/Actuators & Drivers/Drivers/Gate Driver  vHigh=rectifier.s.v_gs_on*1.5 V  vLow=0 V  parameterization=1  rHigh=100 Ohm  rLow=10 Ohm  tRise=20 ns  tFall=20 ns  cLoad=10 nF  enable_faults=0  t_fault=1 s  fault_type=1  uHighValue=0.7  uLowValue=0.3  tHigh=50 ns  tLow=100 ns  ZonTime_specify=off  ZonTime_priority=None  ZonTime=0 s  ZoffTime_specify=off  ZoffTime_priority=None  ZoffTime=0 s  uHigh=2.0 V  uLow=0.8 V
      settings: SourceProductName=Simscape Electronics  SourceProductBaseCode=SN  LogSimulationData=on
  d : PMIOPort  Side=Left
  v_g : PMIOPort  Port=2  Side=Right
  v_s : PMIOPort  Port=3  Side=Right
  connections:
  Gate Driver/LConn2 -- Electrical Reference/LConn1 -- Controlled PWM Voltage/RConn2
  Controlled PWM Voltage/RConn1 -- Gate Driver/LConn1
  v_g/RConn1 -- Gate Driver/RConn1
  v_s/RConn1 -- Gate Driver/RConn2
  d/RConn1 -- Controlled PWM Voltage/LConn1

== system LundellAlternatorDC/Alternator/Armature circuit/Armature circuit (Delta)/i_a sensor ==
  Current Sensor : fl_lib/Electrical/Electrical Sensors/Current Sensor
  PS-Simulink Converter : nesl_utility/PS-Simulink Converter  PhysicalDomain=network_engine_domain  SubClassName=ps_output  LeftPortType=input  RightPortType=output  PseudoPeriodic=off  Frequencies=[]  Unit=1  AffineConversion=off
  + : PMIOPort  Side=Left
  - : PMIOPort  Port=2  Side=Right
  i : Outport
  wires:
  PS-Simulink Converter/1 -> i/1
  connections:
  Current Sensor/RConn2 -- -/RConn1
  Current Sensor/LConn1 -- +/RConn1
  PS-Simulink Converter/LConn1 -- Current Sensor/RConn1

== system LundellAlternatorDC/Alternator/Armature circuit/Armature circuit (Delta)/i_b sensor ==
  Current Sensor : fl_lib/Electrical/Electrical Sensors/Current Sensor
  PS-Simulink Converter : nesl_utility/PS-Simulink Converter  PhysicalDomain=network_engine_domain  SubClassName=ps_output  LeftPortType=input  RightPortType=output  PseudoPeriodic=off  Frequencies=[]  Unit=1  AffineConversion=off
  + : PMIOPort  Side=Left
  - : PMIOPort  Port=2  Side=Right
  i : Outport
  wires:
  PS-Simulink Converter/1 -> i/1
  connections:
  Current Sensor/RConn2 -- -/RConn1
  Current Sensor/LConn1 -- +/RConn1
  PS-Simulink Converter/LConn1 -- Current Sensor/RConn1

== system LundellAlternatorDC/Alternator/Armature circuit/Armature circuit (Delta)/i_c sensor ==
  Current Sensor : fl_lib/Electrical/Electrical Sensors/Current Sensor
  PS-Simulink Converter : nesl_utility/PS-Simulink Converter  PhysicalDomain=network_engine_domain  SubClassName=ps_output  LeftPortType=input  RightPortType=output  PseudoPeriodic=off  Frequencies=[]  Unit=1  AffineConversion=off
  + : PMIOPort  Side=Left
  - : PMIOPort  Port=2  Side=Right
  i : Outport
  wires:
  PS-Simulink Converter/1 -> i/1
  connections:
  Current Sensor/RConn2 -- -/RConn1
  Current Sensor/LConn1 -- +/RConn1
  PS-Simulink Converter/LConn1 -- Current Sensor/RConn1

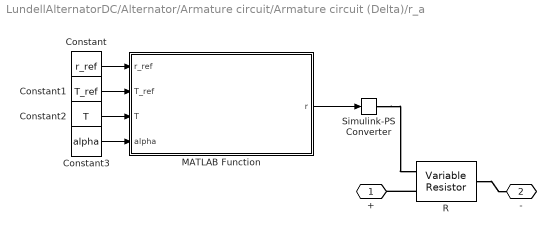
== system LundellAlternatorDC/Alternator/Armature circuit/Armature circuit (Delta)/r_a ==
  Constant : Constant  Value=r_ref
  Constant1 : Constant  Value=T_ref
  Constant2 : Constant  Value=T
  Constant3 : Constant  Value=alpha
  MATLAB Function : MATLAB Function  TreatAsAtomicUnit=on
  R : fl_lib/Electrical/Electrical Elements/Variable Resistor  Rmin=0 Ohm  i_specify=off  i_priority=None  i=0 A  i_nominal_specify=off  i_nominal_unit=A  i_nominal_value=1  v_specify=off  v_priority=None  v=0 V  v_nominal_specify=off  v_nominal_unit=V  v_nominal_value=1
  Simulink-PS Converter : nesl_utility/Simulink-PS Converter  PhysicalDomain=network_engine_domain  SubClassName=ps_input  LeftPortType=input  RightPortType=output  PseudoPeriodic=off  Frequencies=[]  NoiseDistribution=none  NoiseParameters=[]  Unit=1  AffineConversion=off  FilteringAndDerivatives=provide  SimscapeFilterOrder=1  InputFilterTimeConstant=0.001  UdotUserProvided=0
  + : PMIOPort  Side=Left
  - : PMIOPort  Port=2  Side=Right
  wires:
  MATLAB Function/1(r) -> Simulink-PS Converter/1
  Constant/1 -> MATLAB Function/1(r_ref)
  Constant1/1 -> MATLAB Function/2(T_ref)
  Constant3/1 -> MATLAB Function/4(alpha)
  Constant2/1 -> MATLAB Function/3(T)
  connections:
  Simulink-PS Converter/RConn1 -- R/LConn1
  R/RConn1 -- -/RConn1
  R/LConn2 -- +/RConn1

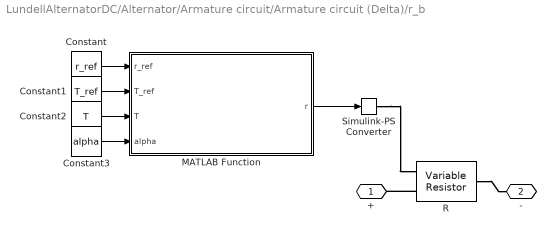
== system LundellAlternatorDC/Alternator/Armature circuit/Armature circuit (Delta)/r_b ==
  Constant : Constant  Value=r_ref
  Constant1 : Constant  Value=T_ref
  Constant2 : Constant  Value=T
  Constant3 : Constant  Value=alpha
  MATLAB Function : MATLAB Function  TreatAsAtomicUnit=on
  R : fl_lib/Electrical/Electrical Elements/Variable Resistor  Rmin=0 Ohm  i_specify=off  i_priority=None  i=0 A  i_nominal_specify=off  i_nominal_unit=A  i_nominal_value=1  v_specify=off  v_priority=None  v=0 V  v_nominal_specify=off  v_nominal_unit=V  v_nominal_value=1
  Simulink-PS Converter : nesl_utility/Simulink-PS Converter  PhysicalDomain=network_engine_domain  SubClassName=ps_input  LeftPortType=input  RightPortType=output  PseudoPeriodic=off  Frequencies=[]  NoiseDistribution=none  NoiseParameters=[]  Unit=1  AffineConversion=off  FilteringAndDerivatives=provide  SimscapeFilterOrder=1  InputFilterTimeConstant=0.001  UdotUserProvided=0
  + : PMIOPort  Side=Left
  - : PMIOPort  Port=2  Side=Right
  wires:
  MATLAB Function/1(r) -> Simulink-PS Converter/1
  Constant/1 -> MATLAB Function/1(r_ref)
  Constant1/1 -> MATLAB Function/2(T_ref)
  Constant3/1 -> MATLAB Function/4(alpha)
  Constant2/1 -> MATLAB Function/3(T)
  connections:
  Simulink-PS Converter/RConn1 -- R/LConn1
  R/RConn1 -- -/RConn1
  R/LConn2 -- +/RConn1

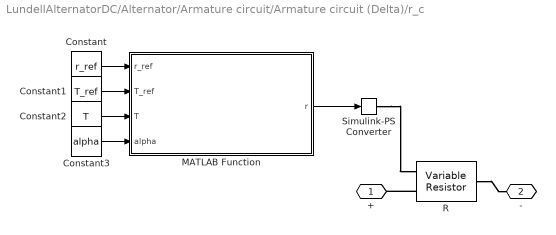
== system LundellAlternatorDC/Alternator/Armature circuit/Armature circuit (Delta)/r_c ==
  Constant : Constant  Value=r_ref
  Constant1 : Constant  Value=T_ref
  Constant2 : Constant  Value=T
  Constant3 : Constant  Value=alpha
  MATLAB Function : MATLAB Function  TreatAsAtomicUnit=on
  R : fl_lib/Electrical/Electrical Elements/Variable Resistor  Rmin=0 Ohm  i_specify=off  i_priority=None  i=0 A  i_nominal_specify=off  i_nominal_unit=A  i_nominal_value=1  v_specify=off  v_priority=None  v=0 V  v_nominal_specify=off  v_nominal_unit=V  v_nominal_value=1
  Simulink-PS Converter : nesl_utility/Simulink-PS Converter  PhysicalDomain=network_engine_domain  SubClassName=ps_input  LeftPortType=input  RightPortType=output  PseudoPeriodic=off  Frequencies=[]  NoiseDistribution=none  NoiseParameters=[]  Unit=1  AffineConversion=off  FilteringAndDerivatives=provide  SimscapeFilterOrder=1  InputFilterTimeConstant=0.001  UdotUserProvided=0
  + : PMIOPort  Side=Left
  - : PMIOPort  Port=2  Side=Right
  wires:
  MATLAB Function/1(r) -> Simulink-PS Converter/1
  Constant/1 -> MATLAB Function/1(r_ref)
  Constant1/1 -> MATLAB Function/2(T_ref)
  Constant3/1 -> MATLAB Function/4(alpha)
  Constant2/1 -> MATLAB Function/3(T)
  connections:
  Simulink-PS Converter/RConn1 -- R/LConn1
  R/RConn1 -- -/RConn1
  R/LConn2 -- +/RConn1

== system LundellAlternatorDC/Alternator/Armature circuit/Armature circuit (Delta)/v_a sensor ==
  PS-Simulink Converter : nesl_utility/PS-Simulink Converter  PhysicalDomain=network_engine_domain  SubClassName=ps_output  LeftPortType=input  RightPortType=output  PseudoPeriodic=off  Frequencies=[]  Unit=1  AffineConversion=off
  Voltage Sensor : fl_lib/Electrical/Electrical Sensors/Voltage Sensor
  + : PMIOPort  Side=Left
  - : PMIOPort  Port=2  Side=Right
  v : Outport
  wires:
  PS-Simulink Converter/1 -> v/1
  connections:
  Voltage Sensor/LConn1 -- +/RConn1
  -/RConn1 -- Voltage Sensor/RConn2
  Voltage Sensor/RConn1 -- PS-Simulink Converter/LConn1

== system LundellAlternatorDC/Alternator/Armature circuit/Armature circuit (Delta)/v_b sensor ==
  PS-Simulink Converter : nesl_utility/PS-Simulink Converter  PhysicalDomain=network_engine_domain  SubClassName=ps_output  LeftPortType=input  RightPortType=output  PseudoPeriodic=off  Frequencies=[]  Unit=1  AffineConversion=off
  Voltage Sensor : fl_lib/Electrical/Electrical Sensors/Voltage Sensor
  + : PMIOPort  Side=Left
  - : PMIOPort  Port=2  Side=Right
  v : Outport
  wires:
  PS-Simulink Converter/1 -> v/1
  connections:
  Voltage Sensor/LConn1 -- +/RConn1
  -/RConn1 -- Voltage Sensor/RConn2
  Voltage Sensor/RConn1 -- PS-Simulink Converter/LConn1

== system LundellAlternatorDC/Alternator/Armature circuit/Armature circuit (Delta)/v_c sensor ==
  PS-Simulink Converter : nesl_utility/PS-Simulink Converter  PhysicalDomain=network_engine_domain  SubClassName=ps_output  LeftPortType=input  RightPortType=output  PseudoPeriodic=off  Frequencies=[]  Unit=1  AffineConversion=off
  Voltage Sensor : fl_lib/Electrical/Electrical Sensors/Voltage Sensor
  + : PMIOPort  Side=Left
  - : PMIOPort  Port=2  Side=Right
  v : Outport
  wires:
  PS-Simulink Converter/1 -> v/1
  connections:
  Voltage Sensor/LConn1 -- +/RConn1
  -/RConn1 -- Voltage Sensor/RConn2
  Voltage Sensor/RConn1 -- PS-Simulink Converter/LConn1

== system LundellAlternatorDC/Alternator/Armature circuit/Armature circuit (Y)/i_a sensor ==
  Current Sensor : fl_lib/Electrical/Electrical Sensors/Current Sensor
  PS-Simulink Converter : nesl_utility/PS-Simulink Converter  PhysicalDomain=network_engine_domain  SubClassName=ps_output  LeftPortType=input  RightPortType=output  PseudoPeriodic=off  Frequencies=[]  Unit=1  AffineConversion=off
  + : PMIOPort  Side=Left
  - : PMIOPort  Port=2  Side=Right
  i : Outport
  wires:
  PS-Simulink Converter/1 -> i/1
  connections:
  Current Sensor/RConn2 -- -/RConn1
  Current Sensor/LConn1 -- +/RConn1
  PS-Simulink Converter/LConn1 -- Current Sensor/RConn1

== system LundellAlternatorDC/Alternator/Armature circuit/Armature circuit (Y)/i_b sensor ==
  Current Sensor : fl_lib/Electrical/Electrical Sensors/Current Sensor
  PS-Simulink Converter : nesl_utility/PS-Simulink Converter  PhysicalDomain=network_engine_domain  SubClassName=ps_output  LeftPortType=input  RightPortType=output  PseudoPeriodic=off  Frequencies=[]  Unit=1  AffineConversion=off
  + : PMIOPort  Side=Left
  - : PMIOPort  Port=2  Side=Right
  i : Outport
  wires:
  PS-Simulink Converter/1 -> i/1
  connections:
  Current Sensor/RConn2 -- -/RConn1
  Current Sensor/LConn1 -- +/RConn1
  PS-Simulink Converter/LConn1 -- Current Sensor/RConn1

== system LundellAlternatorDC/Alternator/Armature circuit/Armature circuit (Y)/i_c sensor ==
  Current Sensor : fl_lib/Electrical/Electrical Sensors/Current Sensor
  PS-Simulink Converter : nesl_utility/PS-Simulink Converter  PhysicalDomain=network_engine_domain  SubClassName=ps_output  LeftPortType=input  RightPortType=output  PseudoPeriodic=off  Frequencies=[]  Unit=1  AffineConversion=off
  + : PMIOPort  Side=Left
  - : PMIOPort  Port=2  Side=Right
  i : Outport
  wires:
  PS-Simulink Converter/1 -> i/1
  connections:
  Current Sensor/RConn2 -- -/RConn1
  Current Sensor/LConn1 -- +/RConn1
  PS-Simulink Converter/LConn1 -- Current Sensor/RConn1

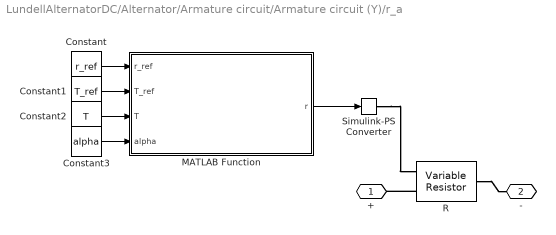
== system LundellAlternatorDC/Alternator/Armature circuit/Armature circuit (Y)/r_a ==
  Constant : Constant  Value=r_ref
  Constant1 : Constant  Value=T_ref
  Constant2 : Constant  Value=T
  Constant3 : Constant  Value=alpha
  MATLAB Function : MATLAB Function  TreatAsAtomicUnit=on
  R : fl_lib/Electrical/Electrical Elements/Variable Resistor  Rmin=0 Ohm  i_specify=off  i_priority=None  i=0 A  i_nominal_specify=off  i_nominal_unit=A  i_nominal_value=1  v_specify=off  v_priority=None  v=0 V  v_nominal_specify=off  v_nominal_unit=V  v_nominal_value=1
  Simulink-PS Converter : nesl_utility/Simulink-PS Converter  PhysicalDomain=network_engine_domain  SubClassName=ps_input  LeftPortType=input  RightPortType=output  PseudoPeriodic=off  Frequencies=[]  NoiseDistribution=none  NoiseParameters=[]  Unit=1  AffineConversion=off  FilteringAndDerivatives=provide  SimscapeFilterOrder=1  InputFilterTimeConstant=0.001  UdotUserProvided=0
  + : PMIOPort  Side=Left
  - : PMIOPort  Port=2  Side=Right
  wires:
  MATLAB Function/1(r) -> Simulink-PS Converter/1
  Constant/1 -> MATLAB Function/1(r_ref)
  Constant1/1 -> MATLAB Function/2(T_ref)
  Constant3/1 -> MATLAB Function/4(alpha)
  Constant2/1 -> MATLAB Function/3(T)
  connections:
  Simulink-PS Converter/RConn1 -- R/LConn1
  R/RConn1 -- -/RConn1
  R/LConn2 -- +/RConn1

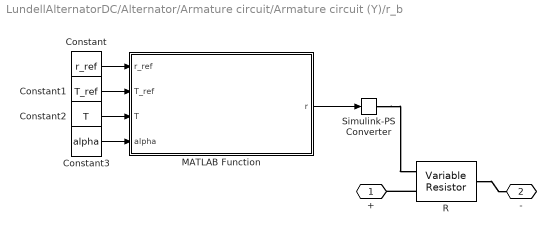
== system LundellAlternatorDC/Alternator/Armature circuit/Armature circuit (Y)/r_b ==
  Constant : Constant  Value=r_ref
  Constant1 : Constant  Value=T_ref
  Constant2 : Constant  Value=T
  Constant3 : Constant  Value=alpha
  MATLAB Function : MATLAB Function  TreatAsAtomicUnit=on
  R : fl_lib/Electrical/Electrical Elements/Variable Resistor  Rmin=0 Ohm  i_specify=off  i_priority=None  i=0 A  i_nominal_specify=off  i_nominal_unit=A  i_nominal_value=1  v_specify=off  v_priority=None  v=0 V  v_nominal_specify=off  v_nominal_unit=V  v_nominal_value=1
  Simulink-PS Converter : nesl_utility/Simulink-PS Converter  PhysicalDomain=network_engine_domain  SubClassName=ps_input  LeftPortType=input  RightPortType=output  PseudoPeriodic=off  Frequencies=[]  NoiseDistribution=none  NoiseParameters=[]  Unit=1  AffineConversion=off  FilteringAndDerivatives=provide  SimscapeFilterOrder=1  InputFilterTimeConstant=0.001  UdotUserProvided=0
  + : PMIOPort  Side=Left
  - : PMIOPort  Port=2  Side=Right
  wires:
  MATLAB Function/1(r) -> Simulink-PS Converter/1
  Constant/1 -> MATLAB Function/1(r_ref)
  Constant1/1 -> MATLAB Function/2(T_ref)
  Constant3/1 -> MATLAB Function/4(alpha)
  Constant2/1 -> MATLAB Function/3(T)
  connections:
  Simulink-PS Converter/RConn1 -- R/LConn1
  R/RConn1 -- -/RConn1
  R/LConn2 -- +/RConn1

== system LundellAlternatorDC/Alternator/Armature circuit/Armature circuit (Y)/r_c ==
  Constant : Constant  Value=r_ref
  Constant1 : Constant  Value=T_ref
  Constant2 : Constant  Value=T
  Constant3 : Constant  Value=alpha
  MATLAB Function : MATLAB Function  TreatAsAtomicUnit=on
  R : fl_lib/Electrical/Electrical Elements/Variable Resistor  Rmin=0 Ohm  i_specify=off  i_priority=None  i=0 A  i_nominal_specify=off  i_nominal_unit=A  i_nominal_value=1  v_specify=off  v_priority=None  v=0 V  v_nominal_specify=off  v_nominal_unit=V  v_nominal_value=1
  Simulink-PS Converter : nesl_utility/Simulink-PS Converter  PhysicalDomain=network_engine_domain  SubClassName=ps_input  LeftPortType=input  RightPortType=output  PseudoPeriodic=off  Frequencies=[]  NoiseDistribution=none  NoiseParameters=[]  Unit=1  AffineConversion=off  FilteringAndDerivatives=provide  SimscapeFilterOrder=1  InputFilterTimeConstant=0.001  UdotUserProvided=0
  + : PMIOPort  Side=Left
  - : PMIOPort  Port=2  Side=Right
  wires:
  MATLAB Function/1(r) -> Simulink-PS Converter/1
  Constant/1 -> MATLAB Function/1(r_ref)
  Constant1/1 -> MATLAB Function/2(T_ref)
  Constant3/1 -> MATLAB Function/4(alpha)
  Constant2/1 -> MATLAB Function/3(T)
  connections:
  Simulink-PS Converter/RConn1 -- R/LConn1
  R/RConn1 -- -/RConn1
  R/LConn2 -- +/RConn1

== system LundellAlternatorDC/Alternator/Armature circuit/Armature circuit (Y)/v_a sensor ==
  PS-Simulink Converter : nesl_utility/PS-Simulink Converter  PhysicalDomain=network_engine_domain  SubClassName=ps_output  LeftPortType=input  RightPortType=output  PseudoPeriodic=off  Frequencies=[]  Unit=1  AffineConversion=off
  Voltage Sensor : fl_lib/Electrical/Electrical Sensors/Voltage Sensor
  + : PMIOPort  Side=Left
  - : PMIOPort  Port=2  Side=Right
  v : Outport
  wires:
  PS-Simulink Converter/1 -> v/1
  connections:
  Voltage Sensor/LConn1 -- +/RConn1
  -/RConn1 -- Voltage Sensor/RConn2
  Voltage Sensor/RConn1 -- PS-Simulink Converter/LConn1

== system LundellAlternatorDC/Alternator/Armature circuit/Armature circuit (Y)/v_b sensor ==
  PS-Simulink Converter : nesl_utility/PS-Simulink Converter  PhysicalDomain=network_engine_domain  SubClassName=ps_output  LeftPortType=input  RightPortType=output  PseudoPeriodic=off  Frequencies=[]  Unit=1  AffineConversion=off
  Voltage Sensor : fl_lib/Electrical/Electrical Sensors/Voltage Sensor
  + : PMIOPort  Side=Left
  - : PMIOPort  Port=2  Side=Right
  v : Outport
  wires:
  PS-Simulink Converter/1 -> v/1
  connections:
  Voltage Sensor/LConn1 -- +/RConn1
  -/RConn1 -- Voltage Sensor/RConn2
  Voltage Sensor/RConn1 -- PS-Simulink Converter/LConn1

== system LundellAlternatorDC/Alternator/Armature circuit/Armature circuit (Y)/v_c sensor ==
  PS-Simulink Converter : nesl_utility/PS-Simulink Converter  PhysicalDomain=network_engine_domain  SubClassName=ps_output  LeftPortType=input  RightPortType=output  PseudoPeriodic=off  Frequencies=[]  Unit=1  AffineConversion=off
  Voltage Sensor : fl_lib/Electrical/Electrical Sensors/Voltage Sensor
  + : PMIOPort  Side=Left
  - : PMIOPort  Port=2  Side=Right
  v : Outport
  wires:
  PS-Simulink Converter/1 -> v/1
  connections:
  Voltage Sensor/LConn1 -- +/RConn1
  -/RConn1 -- Voltage Sensor/RConn2
  Voltage Sensor/RConn1 -- PS-Simulink Converter/LConn1

== matlab function LundellAlternatorDC/Alternator/Armature circuit/Armature circuit (Delta)/r_b/MATLAB Function ==
  data: r_ref input; r output; T_ref input; T input; alpha input
function r = thermalResistance(r_ref, T_ref, T, alpha)

r = r_ref * (1 + alpha * (T - T_ref));

end

== matlab function LundellAlternatorDC/Alternator/Armature circuit/Armature circuit (Delta)/r_a/MATLAB Function ==
  data: r_ref input; r output; T_ref input; T input; alpha input
function r = thermalResistance(r_ref, T_ref, T, alpha)

r = r_ref * (1 + alpha * (T - T_ref));

end

== matlab function LundellAlternatorDC/Alternator/Armature circuit/Armature circuit (Delta)/r_c/MATLAB Function ==
  data: r_ref input; r output; T_ref input; T input; alpha input
function r = thermalResistance(r_ref, T_ref, T, alpha)

r = r_ref * (1 + alpha * (T - T_ref));

end

== matlab function LundellAlternatorDC/Alternator/Armature circuit/Armature circuit (Y)/r_a/MATLAB Function ==
  data: r_ref input; r output; T_ref input; T input; alpha input
function r = thermalResistance(r_ref, T_ref, T, alpha)

r = r_ref * (1 + alpha * (T - T_ref));

end

== matlab function LundellAlternatorDC/Alternator/Armature circuit/Armature circuit (Y)/r_b/MATLAB Function ==
  data: r_ref input; r output; T_ref input; T input; alpha input
function r = thermalResistance(r_ref, T_ref, T, alpha)

r = r_ref * (1 + alpha * (T - T_ref));

end

== matlab function LundellAlternatorDC/Alternator/Armature circuit/Armature circuit (Y)/r_c/MATLAB Function ==
  data: r_ref input; r output; T_ref input; T input; alpha input
function r = thermalResistance(r_ref, T_ref, T, alpha)

r = r_ref * (1 + alpha * (T - T_ref));

end
